simulink model "DKS_datnks"  (R2023b)
settings: Solver=FixedStepDiscrete  StartTime=0.0  StopTime=1.5  FixedStep=1e-7  RelTol=1e-3
values from neighbouring files (symbols this model uses):
  anpha = Vmax^3/(2*Ve*Vmax^2-2*Ve^3)    [datnks.m]
  C = Cmin    [datnks.m]
  Cf = 20e-6    (= 2e-05)    [datnks.m]
  fsw = 10e3    (= 10000)    [datnks.m]
  ki1 = Ve/(sqrt(2)*Pe1)    [datnks.m]
  ki2 = Ve/(sqrt(2)*Pe2)    [datnks.m]
  kv = Vmax/sqrt(2)    [datnks.m]
  L = 1.3e-3    (= 0.0013)    [datnks.m]
  o = 2*anpha    [datnks.m]
  Rf = 0.5    [datnks.m]
  Ts = 1/20000    (= 5e-05)    [datnks.m]
  Ts1 = 1/20000    (= 5e-05)    [datnks.m]
  Udc = 100    [datnks.m]
  wnom = 2*pi*50    (= 314.159265359)    [datnks.m]
undefined symbols (not defined in the file or in its folder): den_nz1, den_nz2, num_nz1, num_nz2
libraries: spsIGBTDiodeLib x8, spsSeriesRLCBranchLib x7, spsCurrentMeasurementLib x6, simulink x6, spsVoltageMeasurementLib x5, spsTriangleGeneratorLib x4, spsBreakerLib x2, spsDCVoltageSourceLib x2, simulink_extras x2, spsSeriesRLCLoadLib x1, dspsrcs4 x1, sps_lib x1
settings Model: SimulationMode=accelerator  Creator=LEGION  LastModifiedBy=Acer
settings SolverCC: ZeroCrossControl=DisableAll  AlgebraicLoopSolver=TrustRegion
settings DataIOCC: ReturnWorkspaceOutputs=off
settings OptimizationCC: ReuseModelBlockBuffer=off
settings DebuggingCC: UnconnectedInputMsg=warning  UnconnectedOutputMsg=warning  UnconnectedLineMsg=warning
settings ModelReferenceCC: EnableRefExpFcnMdlSchedulingChecks=on
settings SFSimCC: CustomCodeUndefinedFunction=UseInterfaceOnly
settings GRTTargetCC: RTWCAPISignals=on  RTWCAPIParams=on

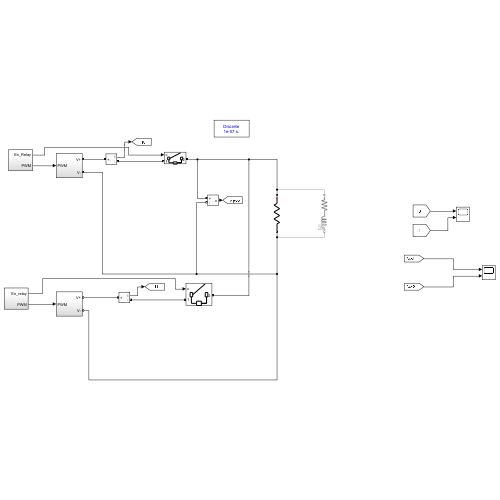
[thumbnail: Simulink's stored preview of the top-level diagram]
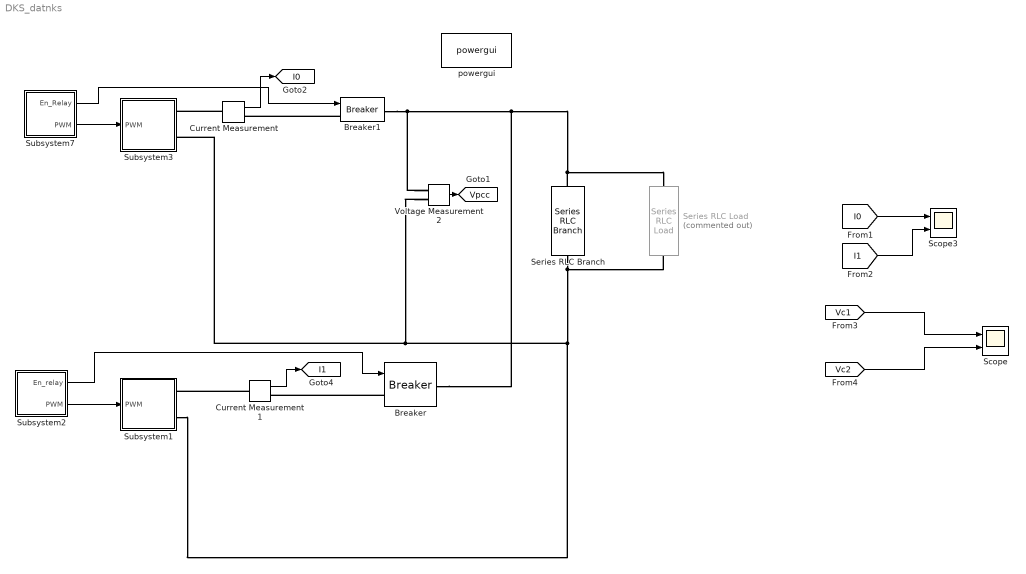
== system DKS_datnks ==
  Breaker : spsBreakerLib/Breaker  InitialState=0  SwitchingTimes="[1/60  5/60]"  External=on  BreakerResistance=0.01  SnubberResistance=1e6  SnubberCapacitance=inf  Measurements=None  MoreParameters=on  NoBreakLoop=off
  Breaker1 : spsBreakerLib/Breaker  InitialState=0  SwitchingTimes="[1/60  5/60]"  External=on  BreakerResistance=0.01  SnubberResistance=1e6  SnubberCapacitance=inf  Measurements=None  MoreParameters=on  NoBreakLoop=off
  Current Measurement : spsCurrentMeasurementLib/Current Measurement  PhasorSimulation=off  OutputType=Complex  PSBequivalent=0
  Current Measurement1 : spsCurrentMeasurementLib/Current Measurement  PhasorSimulation=off  OutputType=Complex  PSBequivalent=0
  Scope : Scope  NumInputPorts=2
  Scope3 : Scope  NumInputPorts=2
  Series RLC Branch : spsSeriesRLCBranchLib/Series RLC Branch  LConnTagsString=__new0  RConnTagsString=__new0  BranchType=R  Resistance=50  Inductance=1e-3  SetiL0=off  InitialCurrent=0  Capacitance=1e-6  Setx0=off  InitialVoltage=0  Measurements=None
  Series RLC Load : spsSeriesRLCLoadLib/Series RLC Load  Commented=on  LConnTagsString=a  RConnTagsString=__new0  NominalVoltage=220  NominalFrequency=50  ActivePower=2550  InductivePower=1850  CapacitivePower=0  Setx0=off  InitialVoltage=0  SetiL0=off  InitialCurrent=0  Measurements=None  LoadType=constant Z
  Subsystem1 : Subsystem
  Subsystem2 : Subsystem
  Subsystem3 : Subsystem
  Subsystem7 : Subsystem
  Voltage Measurement2 : spsVoltageMeasurementLib/Voltage Measurement  PhasorSimulation=off  OutputType=Complex  PSBequivalent=0
  powergui : sps_lib/powergui  Priority=1  SimulationMode=Discrete  SampleTime=1e-7  frequency=60  Iterations=50  frequencyindice=0  Pbase=100e6  ErrMax=1e-4  UnitsV=kV  UnitsW=MW  buscounter=0  FunctionMessages=off  echomessages=off  EnableUseOfTLC=off  CurrentSourceSwitches=off  DisableSnubberDevices=off  DisableRonSwitches=off  DisableVfSwitches=off  DisplayEquations=off  AutomaticDiscreteSolvers=off  SolverType=Tustin/Backward Euler (TBE)  Interpol=off  ExternalGateDelay=off  methode=off  Ts=100  x0status=blocks  SPID=on  SwTol=0  HookPort=off  NonlinearTolerance=1e-4  nMaxIteration=100  ContinueOnMaxIteration=off  RestoreLinks=warning  ResistiveCurrentMeasurement=off  Frange=[0:2:500]  Ylog=off  Xlog=on  ShowGrid=off  save=off  variable=ZData  structure=0  ZoomFFT=off  StartTime=0.0  cycles=1  DisplayStyle=1  fundamental=60  FreqAxis=off  MaxFrequency=1000  frequencyindicesteady=1  RmsSteady=1  display=off
  tag scope: I0=global, I1=global, Vpcc=global
  wires:
  Subsystem7/2(PWM) -> Subsystem3/1("PWM ")
  Current Measurement/1 -> [I0]
  Current Measurement1/1 -> [I1]
  Subsystem2/2(PWM) -> Subsystem1/1("PWM ")
  [I0] -> Scope3/1
  [I1] -> Scope3/2
  Voltage Measurement2/1 -> [Vpcc]
  Subsystem7/1(En_Relay) -> Breaker1/1
  Subsystem2/1(En_relay) -> Breaker/1
  [Vc1] -> Scope/1
  [Vc2] -> Scope/2
  connections:
  Series RLC Branch/LConn1 -- Breaker/RConn1 -- Breaker1/RConn1 -- Voltage Measurement2/LConn1 -- Series RLC Load/LConn1
  Subsystem1/RConn2 -- Series RLC Branch/RConn1 -- Series RLC Load/RConn1 -- Subsystem3/RConn2 -- Voltage Measurement2/LConn2
  Current Measurement/LConn1 -- Subsystem3/RConn1
  Current Measurement1/LConn1 -- Subsystem1/RConn1
  Breaker/LConn1 -- Current Measurement1/RConn1
  Breaker1/LConn1 -- Current Measurement/RConn1

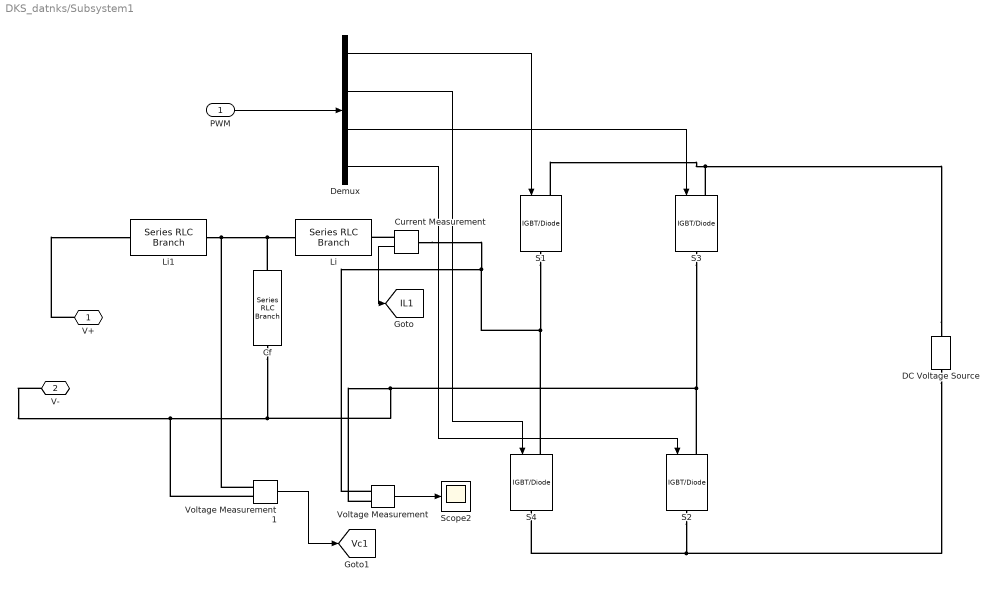
== system DKS_datnks/Subsystem1 ==
  "PWM " : Inport
  "   Cf" : spsSeriesRLCBranchLib/Series RLC Branch  LConnTagsString=__new0  RConnTagsString=__new0  BranchType=C  Resistance=0.1  Inductance=1e-3  SetiL0=off  InitialCurrent=0  Capacitance=Cf  Setx0=off  InitialVoltage=0  Measurements=None
  Current Measurement : spsCurrentMeasurementLib/Current Measurement  PhasorSimulation=off  OutputType=Complex  PSBequivalent=0
  DC Voltage Source : spsDCVoltageSourceLib/DC Voltage Source  Amplitude=Udc  Measurements=None
  Demux : Demux
  Li : spsSeriesRLCBranchLib/Series RLC Branch  LConnTagsString=__new0  RConnTagsString=__new0  BranchType=RL  Resistance=Rf  Inductance=L  SetiL0=off  InitialCurrent=0  Capacitance=1e-6  Setx0=off  InitialVoltage=0  Measurements=None
  Li1 : spsSeriesRLCBranchLib/Series RLC Branch  LConnTagsString=__new0  RConnTagsString=__new0  BranchType=L  Resistance=Rf  Inductance=470e-6  SetiL0=off  InitialCurrent=0  Capacitance=1e-6  Setx0=off  InitialVoltage=0  Measurements=None
  S{1..4} (4 alike) : spsIGBTDiodeLib/IGBT//Diode  Ron=0.001  Rs=1e5  Cs=inf  Measurements=off
  Scope2 : Scope
  Voltage Measurement : spsVoltageMeasurementLib/Voltage Measurement  PhasorSimulation=off  OutputType=Complex  PSBequivalent=0
  Voltage Measurement1 : spsVoltageMeasurementLib/Voltage Measurement  PhasorSimulation=off  OutputType=Complex  PSBequivalent=0
  V+ : PMIOPort  Side=Right
  V- : PMIOPort  Port=2  Side=Right
  tag scope: IL1=global, Vc1=global
  wires:
  "PWM "/1 -> Demux/1
  Demux/1 -> S1/1
  Current Measurement/1 -> [IL1]
  Voltage Measurement/1 -> Scope2/1
  Demux/2 -> S4/1
  Demux/3 -> S3/1
  Demux/4 -> S2/1
  Voltage Measurement1/1 -> [Vc1]
  connections:
  "   Cf"/LConn1 -- Voltage Measurement1/LConn1 -- Li1/RConn1 -- Li/LConn1
  S4/LConn1 -- S1/RConn1 -- Voltage Measurement/LConn1 -- Current Measurement/LConn1
  DC Voltage Source/RConn1 -- S1/LConn1 -- S3/LConn1
  S2/LConn1 -- S3/RConn1 -- Voltage Measurement/LConn2 -- Voltage Measurement1/LConn2 -- V-/RConn1 -- "   Cf"/RConn1
  S2/RConn1 -- DC Voltage Source/LConn1 -- S4/RConn1
  Current Measurement/RConn1 -- Li/RConn1
  V+/RConn1 -- Li1/LConn1

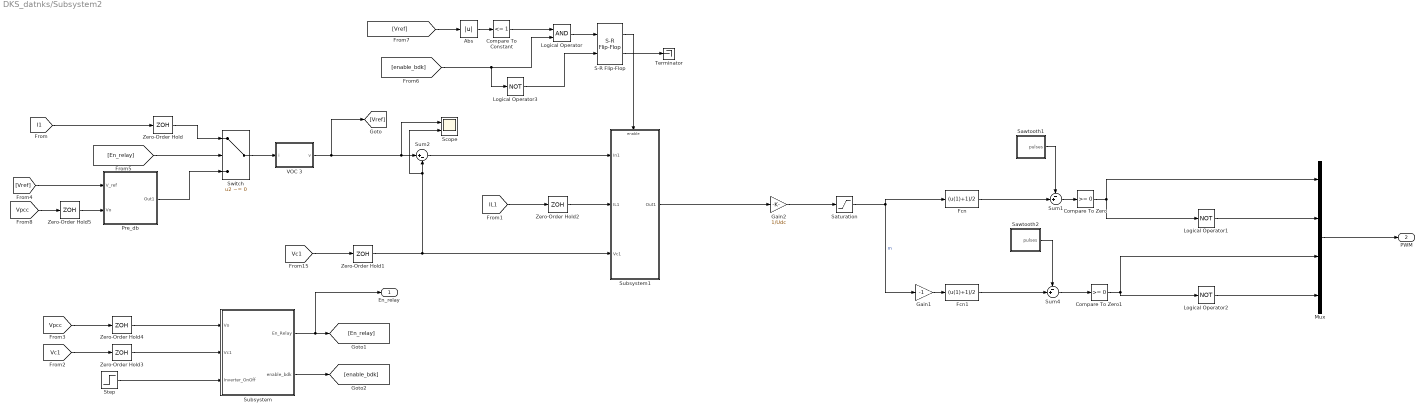
== system DKS_datnks/Subsystem2 ==
  Abs : Abs  SaturateOnIntegerOverflow=off
  Compare To Constant : simulink/Logic and Bit Operations/Compare To Constant  relop=<=  const=1  OutDataTypeStr=boolean
  Compare To Zero : simulink/Logic and Bit Operations/Compare To Zero  relop=>=  OutDataTypeStr=boolean
  Compare To Zero1 : simulink/Logic and Bit Operations/Compare To Zero  relop=>=  OutDataTypeStr=boolean
  Fcn : Fcn  Expr=(u(1)+1)/2
  Fcn1 : Fcn  Expr=(u(1)+1)/2
  Gain1 : Gain  Gain=-1
  Gain2 : Gain  Gain=1/Udc
  Logical Operator : Logic  AllPortsSameDT=off  OutDataTypeStr=boolean
  Logical Operator1 : Logic  Operator=NOT  AllPortsSameDT=off  OutDataTypeStr=boolean
  Logical Operator2 : Logic  Operator=NOT  AllPortsSameDT=off  OutDataTypeStr=boolean
  Logical Operator3 : Logic  Operator=NOT  AllPortsSameDT=off  OutDataTypeStr=boolean
  Mux : Mux
  Pre_db : Subsystem
  S-R Flip-Flop : simulink_extras/Flip Flops/S-R Flip-Flop  initial_condition=0
  Saturation : Saturate  UpperLimit=1  LowerLimit=-1
  Sawtooth1 : Subsystem
  Sawtooth2 : Subsystem
  Scope : Scope  NumInputPorts=2
  Step : Step  Time=0.2  SampleTime=0
  Subsystem : Subsystem
  Subsystem1 : Subsystem
  Sum1 : Sum  Inputs=-+|  InputSameDT=on  SaturateOnIntegerOverflow=on  OutDataTypeStr=Inherit: Same as first input
  Sum2 : Sum  Inputs=|+-
  Sum4 : Sum  Inputs=-+|  InputSameDT=on  SaturateOnIntegerOverflow=on  OutDataTypeStr=Inherit: Same as first input
  Switch : Switch  Criteria=u2 ~= 0  SaturateOnIntegerOverflow=off  InputSameDT=off
  Terminator : Terminator
  VOC 3 : Subsystem
  Zero-Order Hold{,1..5} (6 alike) : ZeroOrderHold  SampleTime=Ts
  En_relay : Outport
  PWM : Outport  Port=2
  wires:
  Mux/1 -> PWM/1
  [Vc1] -> Zero-Order Hold1/1
  Zero-Order Hold1/1 -> Scope/2, Sum2/2, Subsystem1/3(Vc1)
  Sum4/1 -> Compare To Zero1/1
  Fcn/1 -> Sum1/2
  Compare To Zero/1 -> Mux/1, Logical Operator1/1
  Sawtooth2/1(pulses) -> Sum4/1
  Logical Operator2/1 -> Mux/4
  Compare To Zero1/1 -> Mux/3, Logical Operator2/1
  Saturation/1 -> Fcn/1, Gain1/1  "m"
  Fcn1/1 -> Sum4/2
  Gain1/1 -> Fcn1/1
  Sum1/1 -> Compare To Zero/1
  Logical Operator1/1 -> Mux/2
  Sawtooth1/1(pulses) -> Sum1/1
  Gain2/1 -> Saturation/1
  VOC 3/1(v) -> [Vref], Scope/1, Sum2/1
  [I1] -> Zero-Order Hold/1
  Zero-Order Hold3/1 -> Subsystem/2(Vc1)
  [Vc1] -> Zero-Order Hold3/1
  [Vpcc] -> Zero-Order Hold4/1
  Zero-Order Hold4/1 -> Subsystem/1(Vo)
  Step/1 -> Subsystem/3(Inverter_OnOff)
  Subsystem/1(En_Relay) -> En_relay/1, [En_relay]
  [En_relay] -> Switch/2
  Zero-Order Hold/1 -> Switch/1
  Subsystem/2(enable_bdk) -> [enable_bdk]
  Switch/1 -> VOC 3/1(i)
  Sum2/1 -> Subsystem1/1(In1)
  [IL1] -> Zero-Order Hold2/1
  Subsystem1/1(Out1) -> Gain2/1
  Zero-Order Hold2/1 -> Subsystem1/2(IL1)
  [Vref] -> Abs/1
  Abs/1 -> Compare To Constant/1
  Compare To Constant/1 -> Logical Operator/1
  [enable_bdk] -> Logical Operator3/1, Logical Operator/2
  Logical Operator/1 -> S-R Flip-Flop/1
  Logical Operator3/1 -> S-R Flip-Flop/2
  S-R Flip-Flop/1 -> Subsystem1/Enable
  S-R Flip-Flop/2 -> Terminator/1
  [Vref] -> Pre_db/1(V_ref)
  [Vpcc] -> Zero-Order Hold5/1
  Pre_db/1(Out1) -> Switch/3
  Zero-Order Hold5/1 -> Pre_db/2(Vo)

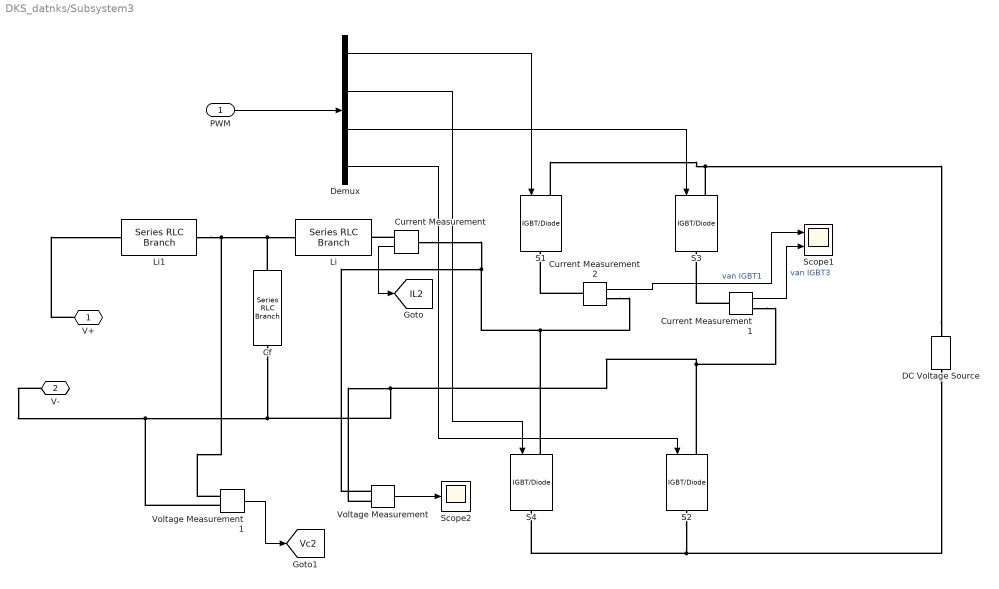
== system DKS_datnks/Subsystem3 ==
  "PWM " : Inport
  "   Cf" : spsSeriesRLCBranchLib/Series RLC Branch  LConnTagsString=__new0  RConnTagsString=__new0  BranchType=C  Resistance=0.1  Inductance=1e-3  SetiL0=off  InitialCurrent=0  Capacitance=Cf  Setx0=off  InitialVoltage=0  Measurements=None
  Current Measurement : spsCurrentMeasurementLib/Current Measurement  PhasorSimulation=off  OutputType=Complex  PSBequivalent=0
  Current Measurement1 : spsCurrentMeasurementLib/Current Measurement  PhasorSimulation=off  OutputType=Complex  PSBequivalent=0
  Current Measurement2 : spsCurrentMeasurementLib/Current Measurement  PhasorSimulation=off  OutputType=Complex  PSBequivalent=0
  DC Voltage Source : spsDCVoltageSourceLib/DC Voltage Source  Amplitude=Udc  Measurements=None
  Demux : Demux
  Li : spsSeriesRLCBranchLib/Series RLC Branch  LConnTagsString=__new0  RConnTagsString=__new0  BranchType=RL  Resistance=Rf  Inductance=L  SetiL0=off  InitialCurrent=0  Capacitance=1e-6  Setx0=off  InitialVoltage=0  Measurements=None
  Li1 : spsSeriesRLCBranchLib/Series RLC Branch  LConnTagsString=__new0  RConnTagsString=__new0  BranchType=L  Resistance=Rf  Inductance=470e-6  SetiL0=off  InitialCurrent=0  Capacitance=1e-6  Setx0=off  InitialVoltage=0  Measurements=None
  S{1..4} (4 alike) : spsIGBTDiodeLib/IGBT//Diode  Ron=0.001  Rs=1e5  Cs=inf  Measurements=off
  Scope1 : Scope  NumInputPorts=2
  Scope2 : Scope
  Voltage Measurement : spsVoltageMeasurementLib/Voltage Measurement  PhasorSimulation=off  OutputType=Complex  PSBequivalent=0
  Voltage Measurement1 : spsVoltageMeasurementLib/Voltage Measurement  PhasorSimulation=off  OutputType=Complex  PSBequivalent=0
  V+ : PMIOPort  Side=Right
  V- : PMIOPort  Port=2  Side=Right
  tag scope: IL2=global, Vc2=global
  wires:
  "PWM "/1 -> Demux/1
  Demux/1 -> S1/1
  Current Measurement/1 -> [IL2]
  Current Measurement1/1 -> Scope1/2  "van IGBT3"
  Voltage Measurement/1 -> Scope2/1
  Current Measurement2/1 -> Scope1/1  "van IGBT1"
  Demux/2 -> S4/1
  Demux/3 -> S3/1
  Demux/4 -> S2/1
  Voltage Measurement1/1 -> [Vc2]
  connections:
  "   Cf"/LConn1 -- Voltage Measurement1/LConn1 -- Li1/RConn1 -- Li/LConn1
  S4/LConn1 -- Current Measurement2/RConn1 -- Voltage Measurement/LConn1 -- Current Measurement/LConn1
  DC Voltage Source/RConn1 -- S1/LConn1 -- S3/LConn1
  S2/LConn1 -- Current Measurement1/RConn1 -- Voltage Measurement/LConn2 -- Voltage Measurement1/LConn2 -- V-/RConn1 -- "   Cf"/RConn1
  S2/RConn1 -- DC Voltage Source/LConn1 -- S4/RConn1
  Current Measurement/RConn1 -- Li/RConn1
  Current Measurement1/LConn1 -- S3/RConn1
  Current Measurement2/LConn1 -- S1/RConn1
  V+/RConn1 -- Li1/LConn1

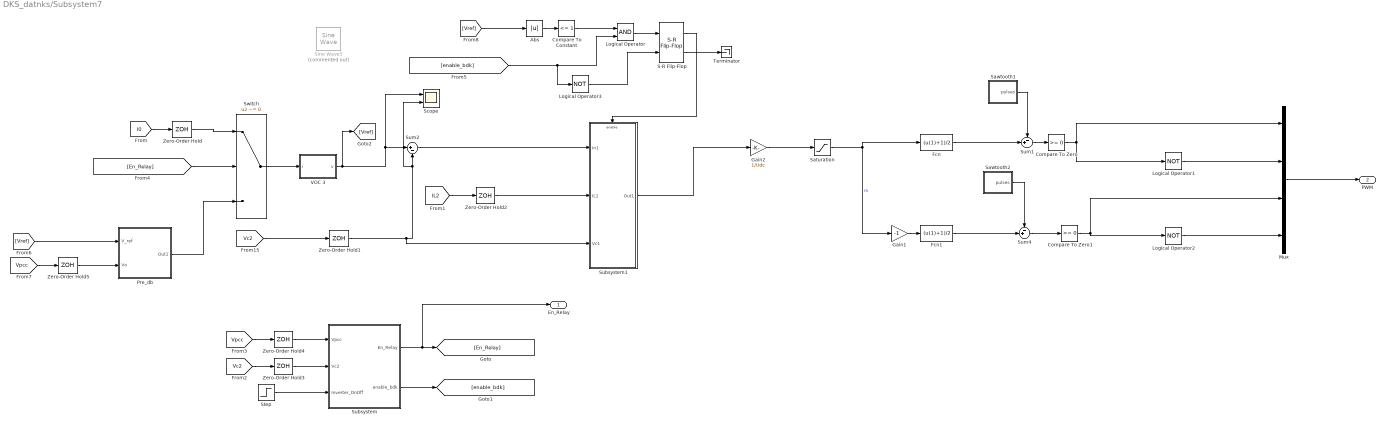
== system DKS_datnks/Subsystem7 ==
  Abs : Abs  SaturateOnIntegerOverflow=off
  Compare To Constant : simulink/Logic and Bit Operations/Compare To Constant  relop=<=  const=1  OutDataTypeStr=boolean
  Compare To Zero : simulink/Logic and Bit Operations/Compare To Zero  relop=>=  OutDataTypeStr=boolean
  Compare To Zero1 : simulink/Logic and Bit Operations/Compare To Zero  relop=>=  OutDataTypeStr=boolean
  Fcn : Fcn  Expr=(u(1)+1)/2
  Fcn1 : Fcn  Expr=(u(1)+1)/2
  Gain1 : Gain  Gain=-1
  Gain2 : Gain  Gain=1/Udc
  Logical Operator : Logic  AllPortsSameDT=off  OutDataTypeStr=boolean
  Logical Operator1 : Logic  Operator=NOT  AllPortsSameDT=off  OutDataTypeStr=boolean
  Logical Operator2 : Logic  Operator=NOT  AllPortsSameDT=off  OutDataTypeStr=boolean
  Logical Operator3 : Logic  Operator=NOT  AllPortsSameDT=off  OutDataTypeStr=boolean
  Mux : Mux
  Pre_db : Subsystem
  S-R Flip-Flop : simulink_extras/Flip Flops/S-R Flip-Flop  initial_condition=0
  Saturation : Saturate  UpperLimit=1  LowerLimit=-1
  Sawtooth1 : Subsystem
  Sawtooth2 : Subsystem
  Scope : Scope  NumInputPorts=2
  Sine Wave5 : dspsrcs4/Sine Wave  Commented=on  Amplitude=60*sqrt(2)  Frequency=50  Phase=0  SampleMode=Discrete  OutComplex=Real  CompMethod=Table lookup  TableSize=Speed  SampleTime=1/100000  SamplesPerFrame=1  ResetState=Restart at time zero  OutputFrames=off  dataType=double  wordLen=32  udDataType=sfix(16)  fracBitsMode=User-defined  numFracBits=24  OutDataTypeStr=double  LastOutDataTypeStr=double
  Step : Step  Time=0.1  SampleTime=0
  Subsystem : Subsystem
  Subsystem1 : Subsystem
  Sum1 : Sum  Inputs=-+|  InputSameDT=on  SaturateOnIntegerOverflow=on  OutDataTypeStr=Inherit: Same as first input
  Sum2 : Sum  Inputs=|+-
  Sum4 : Sum  Inputs=-+|  InputSameDT=on  SaturateOnIntegerOverflow=on  OutDataTypeStr=Inherit: Same as first input
  Switch : Switch  Criteria=u2 ~= 0  SaturateOnIntegerOverflow=off  InputSameDT=off
  Terminator : Terminator
  VOC 3 : Subsystem
  Zero-Order Hold{,1..5} (6 alike) : ZeroOrderHold  SampleTime=Ts
  En_Relay : Outport
  PWM : Outport  Port=2
  wires:
  Mux/1 -> PWM/1
  [IL2] -> Zero-Order Hold2/1
  [Vc2] -> Zero-Order Hold1/1
  Zero-Order Hold1/1 -> Subsystem1/3(Vc1), Scope/2, Sum2/2
  Sum4/1 -> Compare To Zero1/1
  Fcn/1 -> Sum1/2
  Compare To Zero/1 -> Mux/1, Logical Operator1/1
  Sawtooth2/1(pulses) -> Sum4/1
  Logical Operator2/1 -> Mux/4
  Compare To Zero1/1 -> Mux/3, Logical Operator2/1
  Saturation/1 -> Fcn/1, Gain1/1  "m"
  Fcn1/1 -> Sum4/2
  Gain1/1 -> Fcn1/1
  Sum1/1 -> Compare To Zero/1
  Logical Operator1/1 -> Mux/2
  Sawtooth1/1(pulses) -> Sum1/1
  Gain2/1 -> Saturation/1
  [I0] -> Zero-Order Hold/1
  VOC 3/1(v) -> [Vref], Scope/1, Sum2/1
  [Vc2] -> Zero-Order Hold3/1
  Zero-Order Hold3/1 -> Subsystem/2(Vc2)
  Step/1 -> Subsystem/3(Inverter_OnOff)
  Zero-Order Hold4/1 -> Subsystem/1(Vpcc)
  [Vpcc] -> Zero-Order Hold4/1
  Subsystem/1(En_Relay) -> En_Relay/1, [En_Relay]
  Subsystem/2(enable_bdk) -> [enable_bdk]
  [En_Relay] -> Switch/2
  Zero-Order Hold/1 -> Switch/1
  Switch/1 -> VOC 3/1(i)
  [Vpcc] -> Zero-Order Hold5/1
  [Vref] -> Pre_db/1(V_ref)
  Zero-Order Hold5/1 -> Pre_db/2(Vo)
  Sum2/1 -> Subsystem1/1(In1)
  Zero-Order Hold2/1 -> Subsystem1/2(IL1)
  Compare To Constant/1 -> Logical Operator/1
  Abs/1 -> Compare To Constant/1
  Logical Operator/1 -> S-R Flip-Flop/1
  Logical Operator3/1 -> S-R Flip-Flop/2
  [enable_bdk] -> Logical Operator3/1, Logical Operator/2
  [Vref] -> Abs/1
  S-R Flip-Flop/1 -> Subsystem1/Enable
  S-R Flip-Flop/2 -> Terminator/1
  Subsystem1/1(Out1) -> Gain2/1
  Pre_db/1(Out1) -> Switch/3

== system DKS_datnks/Subsystem2/Pre_db ==
  V_ref : Inport
  Vo : Inport  Port=2
  Add : Sum  Inputs=+-
  Constant4 : Constant  Value=10
  Divide : Product  Inputs=*/
  Out1 : Outport
  wires:
  Add/1 -> Divide/1
  Vo/1 -> Add/2
  Constant4/1 -> Divide/2
  Divide/1 -> Out1/1
  V_ref/1 -> Add/1

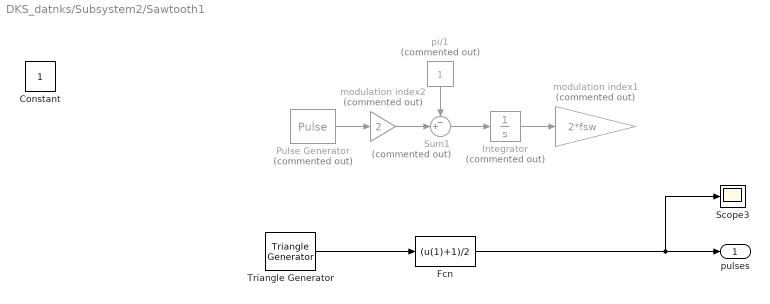
== system DKS_datnks/Subsystem2/Sawtooth1 ==
  Constant : Constant
  Fcn : Fcn  Expr=(u(1)+1)/2
  Integrator : Integrator  Commented=on
  Pulse Generator : DiscretePulseGenerator  Commented=on  PulseType=Time based  Period=1/fsw  PulseWidth=50
  Scope3 : Scope
  Sum1 : Sum  Commented=on  Inputs=-+|  InputSameDT=on  SaturateOnIntegerOverflow=on  OutDataTypeStr=Inherit: Same as first input
  Triangle Generator : spsTriangleGeneratorLib/Triangle Generator  Freq=10e3  Phase=0  Ts=1/(5000*2000)
  modulation index1 : Gain  Commented=on  Gain=2*fsw  SaturateOnIntegerOverflow=on  OutDataTypeStr=Inherit: Same as input  ParamDataTypeStr=Inherit: Same as input
  modulation index2 : Gain  Commented=on  Gain=2  SaturateOnIntegerOverflow=on  OutDataTypeStr=Inherit: Same as input  ParamDataTypeStr=Inherit: Same as input
  pi/1 : Constant  Commented=on
  pulses : Outport  VectorParamsAs1DForOutWhenUnconnected=off
  wires:
  Pulse Generator/1 -> modulation index2/1
  Integrator/1 -> modulation index1/1
  Sum1/1 -> Integrator/1
  modulation index2/1 -> Sum1/2
  pi/1/1 -> Sum1/1
  Triangle Generator/1 -> Fcn/1
  Fcn/1 -> Scope3/1, pulses/1

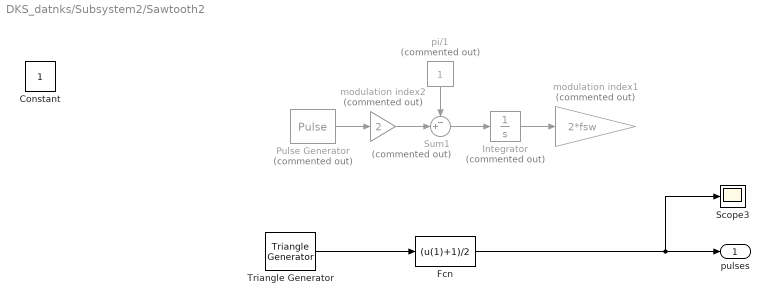
== system DKS_datnks/Subsystem2/Sawtooth2 ==
  Constant : Constant
  Fcn : Fcn  Expr=(u(1)+1)/2
  Integrator : Integrator  Commented=on
  Pulse Generator : DiscretePulseGenerator  Commented=on  PulseType=Time based  Period=1/fsw  PulseWidth=50
  Scope3 : Scope
  Sum1 : Sum  Commented=on  Inputs=-+|  InputSameDT=on  SaturateOnIntegerOverflow=on  OutDataTypeStr=Inherit: Same as first input
  Triangle Generator : spsTriangleGeneratorLib/Triangle Generator  Freq=10e3  Phase=0  Ts=1/(5000*2000)
  modulation index1 : Gain  Commented=on  Gain=2*fsw  SaturateOnIntegerOverflow=on  OutDataTypeStr=Inherit: Same as input  ParamDataTypeStr=Inherit: Same as input
  modulation index2 : Gain  Commented=on  Gain=2  SaturateOnIntegerOverflow=on  OutDataTypeStr=Inherit: Same as input  ParamDataTypeStr=Inherit: Same as input
  pi/1 : Constant  Commented=on
  pulses : Outport  VectorParamsAs1DForOutWhenUnconnected=off
  wires:
  Fcn/1 -> pulses/1, Scope3/1
  Triangle Generator/1 -> Fcn/1
  pi/1/1 -> Sum1/1
  modulation index2/1 -> Sum1/2
  Sum1/1 -> Integrator/1
  Integrator/1 -> modulation index1/1
  Pulse Generator/1 -> modulation index2/1

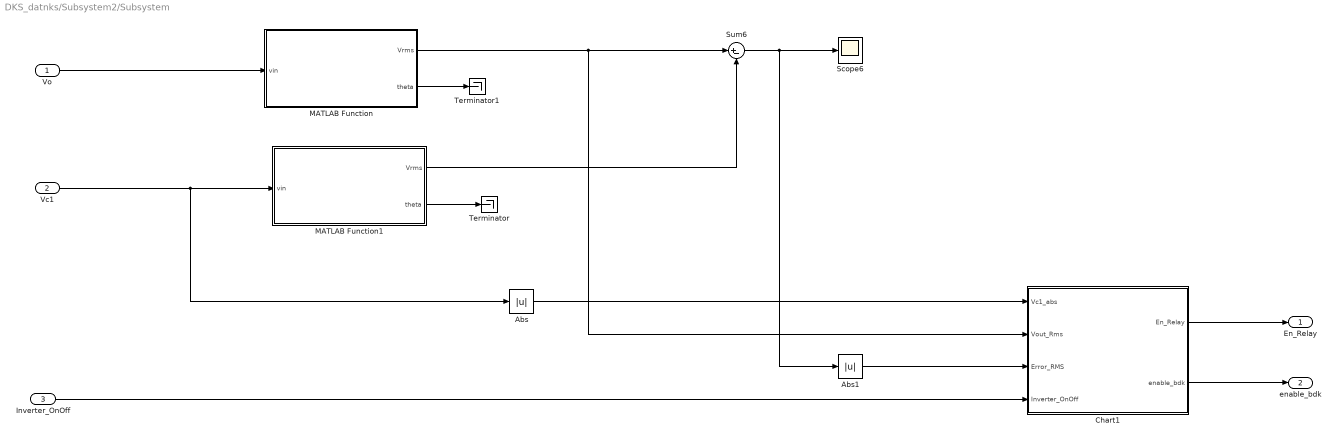
== system DKS_datnks/Subsystem2/Subsystem ==
  Vo : Inport
  Vc1 : Inport  Port=2
  Inverter_OnOff : Inport  Port=3
  Abs : Abs  SaturateOnIntegerOverflow=off
  Abs1 : Abs  SaturateOnIntegerOverflow=off
  Chart1 : Stateflow chart  TreatAsAtomicUnit=on  SystemSampleTime=Ts
      settings: PortSchema="{\"entries\":[{\"content\":{\"sides\":[{\"content\":{\"connectorIds\":[\"In4\",\"In3\",\"In1\",\"In2\"]},\"type\":\"ConnectorPlacement.EquallySpacedRectSide\",\"uuid\":\"a41d96ef-4339-445d-adf1-46a375c1ebfc\"},{\"content\":{\"connectorIds\":[\"Out1\",\"Out2\"],\"side\":\"RIGHT\"},\"type\":\"ConnectorPlacement.EquallySpacedRectSide\",\"uuid\":\"433b8e1f-da11-4860-b5b3-686501ffdddb\"},{\"content\":{\"side\":\"TOP\"},\"type\":\"ConnectorPlacement.EquallySpacedRectSide\",\"uuid\":\"a76241af-ec7f-4a92-ba0a-9793b7afdcf0\"}]},\"type\":\"ConnectorPlacement.EquallySpacedConnector\",\"uuid\":\"1de099f0-7c57-4924-8764-8a627297889a\"}],\"packageUris\":[\"http://schema.mathworks.com/mf0/Connector/R2020b\"],\"version\":\"1.0\"}"
  MATLAB Function : MATLAB Function  TreatAsAtomicUnit=on
  MATLAB Function1 : MATLAB Function  TreatAsAtomicUnit=on
  Scope6 : Scope
  Sum6 : Sum  Inputs=|+-
  Terminator : Terminator
  Terminator1 : Terminator
  En_Relay : Outport
  enable_bdk : Outport  Port=2
  wires:
  MATLAB Function/1(Vrms) -> Chart1/3(Vout_Rms), Sum6/1
  MATLAB Function1/2(theta) -> Terminator/1
  MATLAB Function/2(theta) -> Terminator1/1
  MATLAB Function1/1(Vrms) -> Sum6/2
  Abs1/1 -> Chart1/1(Error_RMS)
  Vc1/1 -> Abs/1, MATLAB Function1/1(vin)
  Sum6/1 -> Abs1/1, Scope6/1
  Abs/1 -> Chart1/4(Vc1_abs)
  Inverter_OnOff/1 -> Chart1/2(Inverter_OnOff)
  Chart1/1(En_Relay) -> En_Relay/1
  Vo/1 -> MATLAB Function/1(vin)
  Chart1/2(enable_bdk) -> enable_bdk/1

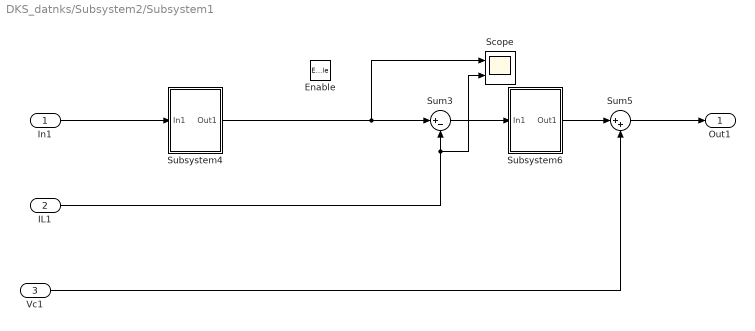
== system DKS_datnks/Subsystem2/Subsystem1 ==
  In1 : Inport
  IL1 : Inport  Port=2
  Vc1 : Inport  Port=3
  Enable : EnablePort  StatesWhenEnabling=reset
  Scope : Scope  NumInputPorts=2
  Subsystem4 : Subsystem
  Subsystem6 : Subsystem
  Sum3 : Sum  Inputs=|+-
  Sum5 : Sum  Inputs=|++
  Out1 : Outport  OutputWhenDisabled=reset  InitialOutput=[0]
  wires:
  Sum5/1 -> Out1/1
  Sum3/1 -> Subsystem6/1(In1)
  IL1/1 -> Scope/2, Sum3/2
  Subsystem6/1(Out1) -> Sum5/1
  In1/1 -> Subsystem4/1(In1)
  Subsystem4/1(Out1) -> Scope/1, Sum3/1
  Vc1/1 -> Sum5/2

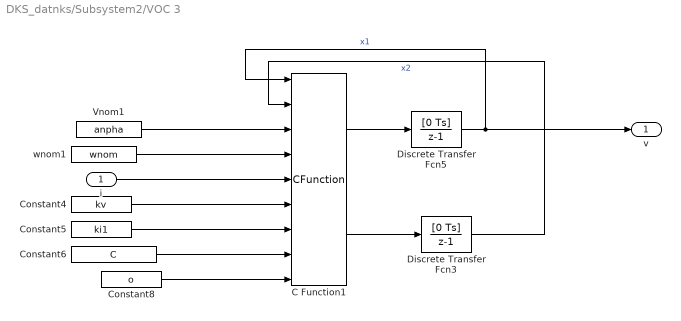
== system DKS_datnks/Subsystem2/VOC 3 ==
  i : Inport
  C Function1 : CFunction  OutputCode=|  SampleTime=Ts
      | y1 = (kv*kv*o/anpha-u1*u1-u2*u2)*u1*anpha/(C*kv*kv)-wnom*u2-ki*kv*i/C;
      | y2 = wnom*u1;
  Constant4 : Constant  Value=kv  OutDataTypeStr=double  SampleTime=-1
  Constant5 : Constant  Value=ki1  OutDataTypeStr=double  SampleTime=-1
  Constant6 : Constant  Value=C  OutDataTypeStr=double  SampleTime=-1
  Constant8 : Constant  Value=o  OutDataTypeStr=double  SampleTime=-1
  Discrete Transfer Fcn3 : DiscreteTransferFcn  Numerator=[0 Ts]  Denominator=[1 -1]  SampleTime=Ts1
  Discrete Transfer Fcn5 : DiscreteTransferFcn  Numerator=[0 Ts]  Denominator=[1 -1]  SampleTime=Ts1
  Vnom1 : Constant  Value=anpha  OutDataTypeStr=double  SampleTime=-1
  wnom1 : Constant  Value=wnom  OutDataTypeStr=double  SampleTime=-1
  v : Outport
  wires:
  Discrete Transfer Fcn5/1 -> C Function1/1, v/1  "x1"
  C Function1/1 -> Discrete Transfer Fcn5/1
  Vnom1/1 -> C Function1/3
  Constant8/1 -> C Function1/9
  Constant4/1 -> C Function1/6
  Constant6/1 -> C Function1/8
  C Function1/2 -> Discrete Transfer Fcn3/1
  wnom1/1 -> C Function1/4
  Constant5/1 -> C Function1/7
  Discrete Transfer Fcn3/1 -> C Function1/2  "x2"
  i/1 -> C Function1/5

== system DKS_datnks/Subsystem7/Pre_db ==
  V_ref : Inport
  Vo : Inport  Port=2
  Add : Sum  Inputs=+-
  Constant4 : Constant  Value=10
  Divide : Product  Inputs=*/
  Out1 : Outport
  wires:
  Add/1 -> Divide/1
  Vo/1 -> Add/2
  Constant4/1 -> Divide/2
  Divide/1 -> Out1/1
  V_ref/1 -> Add/1

== system DKS_datnks/Subsystem7/Sawtooth1 ==
  Fcn : Fcn  Expr=(u(1)+1)/2
  Triangle Generator : spsTriangleGeneratorLib/Triangle Generator  Freq=10e3  Phase=0  Ts=1/(5000*2000)
  pulses : Outport  VectorParamsAs1DForOutWhenUnconnected=off
  wires:
  Fcn/1 -> pulses/1
  Triangle Generator/1 -> Fcn/1

== system DKS_datnks/Subsystem7/Sawtooth2 ==
  Fcn : Fcn  Expr=(u(1)+1)/2
  Triangle Generator : spsTriangleGeneratorLib/Triangle Generator  Freq=10e3  Phase=0  Ts=1/(5000*2000)
  pulses : Outport  VectorParamsAs1DForOutWhenUnconnected=off
  wires:
  Triangle Generator/1 -> Fcn/1
  Fcn/1 -> pulses/1

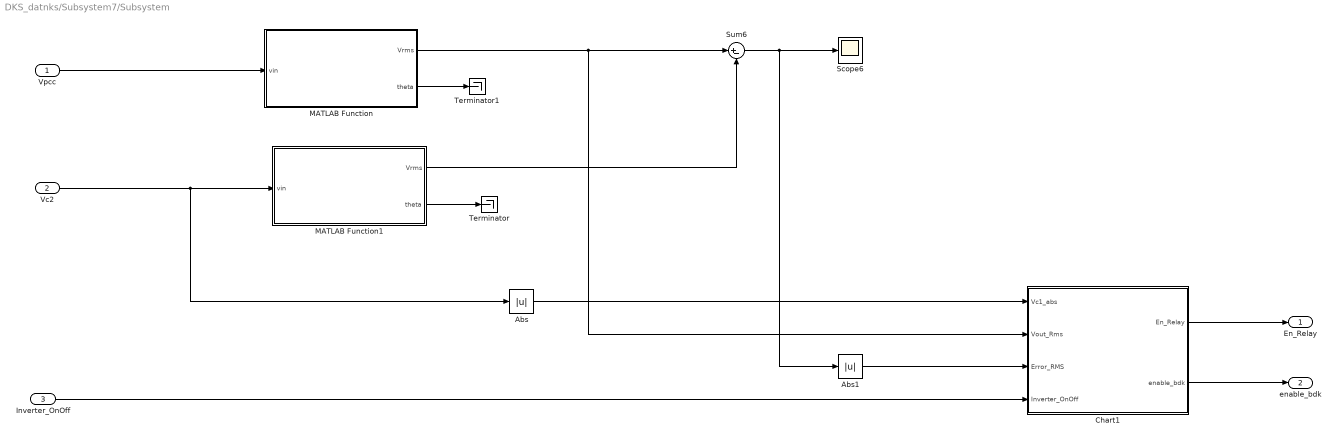
== system DKS_datnks/Subsystem7/Subsystem ==
  Vpcc : Inport
  Vc2 : Inport  Port=2
  Inverter_OnOff : Inport  Port=3
  Abs : Abs  SaturateOnIntegerOverflow=off
  Abs1 : Abs  SaturateOnIntegerOverflow=off
  Chart1 : Stateflow chart  TreatAsAtomicUnit=on  SystemSampleTime=Ts
      settings: PortSchema="{\"entries\":[{\"content\":{\"sides\":[{\"content\":{\"connectorIds\":[\"In4\",\"In3\",\"In1\",\"In2\"]},\"type\":\"ConnectorPlacement.EquallySpacedRectSide\",\"uuid\":\"a41d96ef-4339-445d-adf1-46a375c1ebfc\"},{\"content\":{\"connectorIds\":[\"Out1\",\"Out2\"],\"side\":\"RIGHT\"},\"type\":\"ConnectorPlacement.EquallySpacedRectSide\",\"uuid\":\"433b8e1f-da11-4860-b5b3-686501ffdddb\"},{\"content\":{\"side\":\"TOP\"},\"type\":\"ConnectorPlacement.EquallySpacedRectSide\",\"uuid\":\"a76241af-ec7f-4a92-ba0a-9793b7afdcf0\"}]},\"type\":\"ConnectorPlacement.EquallySpacedConnector\",\"uuid\":\"1de099f0-7c57-4924-8764-8a627297889a\"}],\"packageUris\":[\"http://schema.mathworks.com/mf0/Connector/R2020b\"],\"version\":\"1.0\"}"
  MATLAB Function : MATLAB Function  TreatAsAtomicUnit=on
  MATLAB Function1 : MATLAB Function  TreatAsAtomicUnit=on
  Scope6 : Scope
  Sum6 : Sum  Inputs=|+-
  Terminator : Terminator
  Terminator1 : Terminator
  En_Relay : Outport
  enable_bdk : Outport  Port=2
  wires:
  MATLAB Function/1(Vrms) -> Chart1/3(Vout_Rms), Sum6/1
  MATLAB Function1/2(theta) -> Terminator/1
  MATLAB Function/2(theta) -> Terminator1/1
  MATLAB Function1/1(Vrms) -> Sum6/2
  Abs1/1 -> Chart1/1(Error_RMS)
  Vc2/1 -> Abs/1, MATLAB Function1/1(vin)
  Sum6/1 -> Abs1/1, Scope6/1
  Abs/1 -> Chart1/4(Vc1_abs)
  Inverter_OnOff/1 -> Chart1/2(Inverter_OnOff)
  Chart1/1(En_Relay) -> En_Relay/1
  Vpcc/1 -> MATLAB Function/1(vin)
  Chart1/2(enable_bdk) -> enable_bdk/1

== system DKS_datnks/Subsystem7/Subsystem1 ==
  In1 : Inport
  IL1 : Inport  Port=2
  Vc1 : Inport  Port=3
  Enable : EnablePort  StatesWhenEnabling=reset
  Scope : Scope  NumInputPorts=2
  Subsystem4 : Subsystem
  Subsystem6 : Subsystem
  Sum3 : Sum  Inputs=|+-
  Sum5 : Sum  Inputs=|++
  Out1 : Outport  OutputWhenDisabled=reset  InitialOutput=[0]
  wires:
  Sum5/1 -> Out1/1
  Sum3/1 -> Subsystem6/1(In1)
  IL1/1 -> Scope/2, Sum3/2
  Subsystem6/1(Out1) -> Sum5/1
  In1/1 -> Subsystem4/1(In1)
  Subsystem4/1(Out1) -> Scope/1, Sum3/1
  Vc1/1 -> Sum5/2

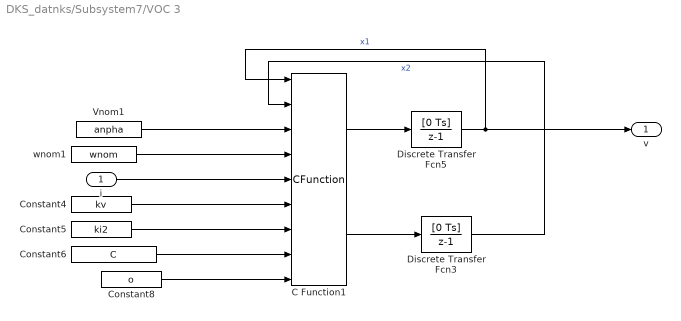
== system DKS_datnks/Subsystem7/VOC 3 ==
  i : Inport
  C Function1 : CFunction  OutputCode=|  SampleTime=Ts
      | y1 = (kv*kv*o/anpha-u1*u1-u2*u2)*u1*anpha/(C*kv*kv)-wnom*u2-ki*kv*i/C;
      | y2 = wnom*u1;
  Constant4 : Constant  Value=kv  OutDataTypeStr=double  SampleTime=-1
  Constant5 : Constant  Value=ki2  OutDataTypeStr=double  SampleTime=-1
  Constant6 : Constant  Value=C  OutDataTypeStr=double  SampleTime=-1
  Constant8 : Constant  Value=o  OutDataTypeStr=double  SampleTime=-1
  Discrete Transfer Fcn3 : DiscreteTransferFcn  Numerator=[0 Ts]  Denominator=[1 -1]  SampleTime=Ts1
  Discrete Transfer Fcn5 : DiscreteTransferFcn  Numerator=[0 Ts]  Denominator=[1 -1]  SampleTime=Ts1
  Vnom1 : Constant  Value=anpha  OutDataTypeStr=double  SampleTime=-1
  wnom1 : Constant  Value=wnom  OutDataTypeStr=double  SampleTime=-1
  v : Outport
  wires:
  Discrete Transfer Fcn5/1 -> C Function1/1, v/1  "x1"
  C Function1/1 -> Discrete Transfer Fcn5/1
  Vnom1/1 -> C Function1/3
  Constant8/1 -> C Function1/9
  Constant4/1 -> C Function1/6
  Constant6/1 -> C Function1/8
  C Function1/2 -> Discrete Transfer Fcn3/1
  wnom1/1 -> C Function1/4
  Constant5/1 -> C Function1/7
  Discrete Transfer Fcn3/1 -> C Function1/2  "x2"
  i/1 -> C Function1/5

== system DKS_datnks/Subsystem2/Subsystem1/Subsystem4 ==
  In1 : Inport
  Discrete Transfer Fcn1 : DiscreteTransferFcn  Commented=on  Numerator=[num_nz2]  Denominator=[den_nz2]  SampleTime=Ts1
  Discrete Transfer Fcn8 : DiscreteTransferFcn  Numerator=[num_nz2]  Denominator=[den_nz2]  SampleTime=Ts
  Out1 : Outport
  wires:
  In1/1 -> Discrete Transfer Fcn8/1
  Discrete Transfer Fcn8/1 -> Out1/1

== system DKS_datnks/Subsystem2/Subsystem1/Subsystem6 ==
  In1 : Inport  OutDataTypeStr=double
  Discrete Transfer Fcn8 : DiscreteTransferFcn  Numerator=[num_nz1]  Denominator=[den_nz1]  SampleTime=Ts
  Out1 : Outport  OutDataTypeStr=double
  wires:
  In1/1 -> Discrete Transfer Fcn8/1
  Discrete Transfer Fcn8/1 -> Out1/1

== system DKS_datnks/Subsystem7/Subsystem1/Subsystem4 ==
  In1 : Inport
  Discrete Transfer Fcn1 : DiscreteTransferFcn  Commented=on  Numerator=[num_nz2]  Denominator=[den_nz2]  SampleTime=Ts1
  Discrete Transfer Fcn8 : DiscreteTransferFcn  Numerator=[num_nz2]  Denominator=[den_nz2]  SampleTime=Ts
  Out1 : Outport
  wires:
  In1/1 -> Discrete Transfer Fcn8/1
  Discrete Transfer Fcn8/1 -> Out1/1

== system DKS_datnks/Subsystem7/Subsystem1/Subsystem6 ==
  In1 : Inport  OutDataTypeStr=double
  Discrete Transfer Fcn8 : DiscreteTransferFcn  Numerator=[num_nz1]  Denominator=[den_nz1]  SampleTime=Ts
  Out1 : Outport  OutDataTypeStr=double
  wires:
  In1/1 -> Discrete Transfer Fcn8/1
  Discrete Transfer Fcn8/1 -> Out1/1

== stateflow chart DKS_datnks/Subsystem2/Subsystem/Chart1 ==
  state Off
    En_Relay = false;
    enable_bdk = false;
    if (Vout_Rms < 10)
    Grid_Off = Grid_Off + 1;
    Grid_On = 0;
    else
    Grid_On = Grid_On + 1;
    Grid_Off = 0;
    end
  state On_Normal
    En_Relay = true;
    enable_bdk = true;
  state Pre_Synchronous
    En_Relay = false;
    enable_bdk = true;
    if (Error_RMS < 5)
    Change_status = Change_status+1;
    else
    Change_status = 0;
    end
  (default) -> Off
  Off -> On_Normal [order 1] : [Inverter_OnOff == true && Grid_Off >1000]
  On_Normal -> Off : [Inverter_OnOff == false]
  Off -> Pre_Synchronous [order 2] : [Inverter_OnOff == true && Grid_On >1000]
  Pre_Synchronous -> Off [order 2] : [Inverter_OnOff == false]
  Pre_Synchronous -> On_Normal [order 1] : [Change_status > 1000 && Vc1_abs < 10]
  data: Error_RMS input; Inverter_OnOff input; Vout_Rms input; Vc1_abs input; En_Relay output =false; Change_status local =0; Grid_Off local =0; Grid_On local =0; enable_bdk output boolean

== matlab function DKS_datnks/Subsystem2/Subsystem/MATLAB Function ==
  data: vin input; Vrms output; theta output
function [Vrms, theta] = single_phase_rms_phase(vin)
%#codegen

persistent v_alpha v_beta
persistent k w Ts

if isempty(v_alpha)
    v_alpha = 0;
    v_beta  = 0;
    
    Ts = 0.5e-4;          % sampling time (10 kHz -> sửa theo bạn)
    w  = 2*pi*50;       % tần số danh định 50Hz
    k  = sqrt(2);       % gain SOGI
end

% ---- SOGI ----
e = vin - v_alpha;

v_alpha = v_alpha + Ts*( k*w*e - w*v_beta );
v_beta  = v_beta  + Ts*( w*v_alpha );

% ---- RMS ----
Vrms = sqrt( (v_alpha*v_alpha + v_beta*v_beta)/2 );

% ---- Phase ----
theta = atan2(v_beta , v_alpha);

end

== matlab function DKS_datnks/Subsystem2/Subsystem/MATLAB Function1 ==
  data: vin input; Vrms output; theta output
function [Vrms, theta] = single_phase_rms_phase(vin)
%#codegen

persistent v_alpha v_beta
persistent k w Ts

if isempty(v_alpha)
    v_alpha = 0;
    v_beta  = 0;
    
    Ts = 0.5e-4;          % sampling time (10 kHz -> sửa theo bạn)
    w  = 2*pi*50;       % tần số danh định 50Hz
    k  = sqrt(2);       % gain SOGI
end

% ---- SOGI ----
e = vin - v_alpha;

v_alpha = v_alpha + Ts*( k*w*e - w*v_beta );
v_beta  = v_beta  + Ts*( w*v_alpha );

% ---- RMS ----
Vrms = sqrt( (v_alpha*v_alpha + v_beta*v_beta)/2 );

% ---- Phase ----
theta = atan2(v_beta , v_alpha);

end

== matlab function DKS_datnks/Subsystem7/Subsystem/MATLAB Function ==
  data: vin input; Vrms output; theta output
function [Vrms, theta] = single_phase_rms_phase(vin)
%#codegen

persistent v_alpha v_beta
persistent k w Ts

if isempty(v_alpha)
    v_alpha = 0;
    v_beta  = 0;
    
    Ts = 0.5e-4;          % sampling time (10 kHz -> sửa theo bạn)
    w  = 2*pi*50;       % tần số danh định 50Hz
    k  = sqrt(2);       % gain SOGI
end

% ---- SOGI ----
e = vin - v_alpha;

v_alpha = v_alpha + Ts*( k*w*e - w*v_beta );
v_beta  = v_beta  + Ts*( w*v_alpha );

% ---- RMS ----
Vrms = sqrt( (v_alpha*v_alpha + v_beta*v_beta)/2 );

% ---- Phase ----
theta = atan2(v_beta , v_alpha);

end

== matlab function DKS_datnks/Subsystem7/Subsystem/MATLAB Function1 ==
  data: vin input; Vrms output; theta output
function [Vrms, theta] = single_phase_rms_phase(vin)
%#codegen

persistent v_alpha v_beta
persistent k w Ts

if isempty(v_alpha)
    v_alpha = 0;
    v_beta  = 0;
    
    Ts = 0.5e-4;          % sampling time (10 kHz -> sửa theo bạn)
    w  = 2*pi*50;       % tần số danh định 50Hz
    k  = sqrt(2);       % gain SOGI
end

% ---- SOGI ----
e = vin - v_alpha;

v_alpha = v_alpha + Ts*( k*w*e - w*v_beta );
v_beta  = v_beta  + Ts*( w*v_alpha );

% ---- RMS ----
Vrms = sqrt( (v_alpha*v_alpha + v_beta*v_beta)/2 );

% ---- Phase ----
theta = atan2(v_beta , v_alpha);

end

== stateflow chart DKS_datnks/Subsystem7/Subsystem/Chart1 ==
  state Off
    En_Relay = false;
    enable_bdk = false;
    if (Vout_Rms < 10)
    Grid_Off = Grid_Off + 1;
    Grid_On = 0;
    else
    Grid_On = Grid_On + 1;
    Grid_Off = 0;
    end
  state On_Normal
    En_Relay = true;
    enable_bdk = true;
  state Pre_Synchronous
    En_Relay = false;
    enable_bdk = true;
    if (Error_RMS < 5)
    Change_status = Change_status+1;
    else
    Change_status = 0;
    end
  (default) -> Off
  Off -> On_Normal [order 1] : [Inverter_OnOff == true && Grid_Off >1000]
  On_Normal -> Off : [Inverter_OnOff == false]
  Off -> Pre_Synchronous [order 2] : [Inverter_OnOff == true && Grid_On >1000]
  Pre_Synchronous -> Off [order 2] : [Inverter_OnOff == false]
  Pre_Synchronous -> On_Normal [order 1] : [Change_status > 1000 && Vc1_abs < 10]
  data: Error_RMS input; Inverter_OnOff input; Vout_Rms input; Vc1_abs input; En_Relay output =false; Change_status local =0; Grid_Off local =0; Grid_On local =0; enable_bdk output boolean
